simulink model "Controller_HIL"  (R2024a)
settings: Solver=FixedStepDiscrete  StartTime=0.0  StopTime=inf  FixedStep=ts_controller  RelTol=1e-3
InitFcn:
  | mbd_s32k_consistency_checks(bdroot(gcs));
undefined symbols (not defined in the file): Battery, BMS_Controller_State, Charging_State, currentFactor, CV_Gain, DiscIntNeverNeededParam, I_cc, LQFP, MaxCellVoltThrsld, noCurrent, Ns_Module, NumModules, OverCellVoltageLimit, SOCInit, SRE, ts_controller, ts_system, UnderCellVoltageLimit, voltThreshold
libraries: mbd_s32k1xx_ec_toolbox x104, etargetslib x95, mbd_bcc_ec_toolbox x30, hdlsllib x11, simulink x6, sharedTrackingLibrary x2
(part 1 of 4)
settings Model: DataDictionary=VTOLDynamicsData.sldd  EnableAccessToBaseWorkspace=off  Creator=vasileios.amoiridis  LastModifiedBy=jatin.anand
settings DataIOCC: ExternalInput=off  InitialState=off  SaveOutput=off  SignalLogging=off  SaveTime=off
settings OptimizationCC: DefaultParameterBehavior=Inlined  DefaultUnderspecifiedDataType=single  EnhancedBackFolding=on  PassReuseOutputArgsAs=Individual arguments  ZeroExternalMemoryAtStartup=off  ZeroInternalMemoryAtStartup=off  OptimizeBlockOrder=speed  DifferentSizesBufferReuse=on  OptimizationCustomize=off  EfficientTunableParamExpr=on
settings DebuggingCC: InheritedTsInSrcMsg=none  SingleTaskRateTransMsg=error  ParameterTunabilityLossMsg=error  UnconnectedInputMsg=error  UnconnectedOutputMsg=error  UnconnectedLineMsg=error  UnknownTsInhSupMsg=error
settings HardwareCC: ProdBitPerPointer=32  ProdBitPerSizeT=32  ProdBitPerPtrDiffT=32  ProdLargestAtomicInteger=Long  ProdLargestAtomicFloat=Double  ProdWordSize=32  ProdHWDeviceType=ARM Compatible->ARM Cortex
settings SFSimCC: MATLABDynamicMemAlloc=off
settings RTWCC: Description=Model Based Design Toolbox S32K1xx Code Generation Target  SystemTargetFile=mbd_s32k.tlc  MakeCommand=mbd_s32k_make_rtw COPY_MDLREF_INCLUDES=0  TemplateMakefile=mbd_s32k.tmf  GPUComputeCapability=3.5
settings CodeAppCC: ForceParamTrailComments=on  IgnoreCustomStorageClasses=off  OperatorAnnotations=on  SimulinkDataObjDesc=on  SFDataObjDesc=on  InsertBlockDesc=on
settings STFCustomTargetCC: MultiwordLength=256  CombineOutputUpdateFcns=on  ERTCustomFileBanners=on  SupportContinuousTime=off  SupportNonInlinedSFcns=off  RemoveResetFunc=on  MATLABClassNameForMDSCustomization=Simulink.SoftwareTarget.ERTCustomization  GRTInterface=off  UseToolchainInfoCompliant=off  SystemTargetFile=mbd_s32k.tlc
settings ERTTargetCC: TargetLangStandard=C99 (ISO)  ParMdlRefBuildCompliant=off  CompOptLevelCompliant=off  ConcurrentExecutionCompliant=off  ModelStepFunctionPrototypeControlCompliant=off  CPPClassGenCompliant=off  UseToolchainInfoCompliant=off  InlinedParameterPlacement=NonHierarchical  ERTSrcFileBannerTemplate=mbd_ert_code_template.cgt  ERTHdrFileBannerTemplate=mbd_ert_code_template.cgt  ERTDataSrcFileTemplate=mbd_ert_code_template.cgt  ERTDataHdrFileTemplate=mbd_ert_code_template.cgt  ERTCustomFileTemplate=example_file_process.tlc

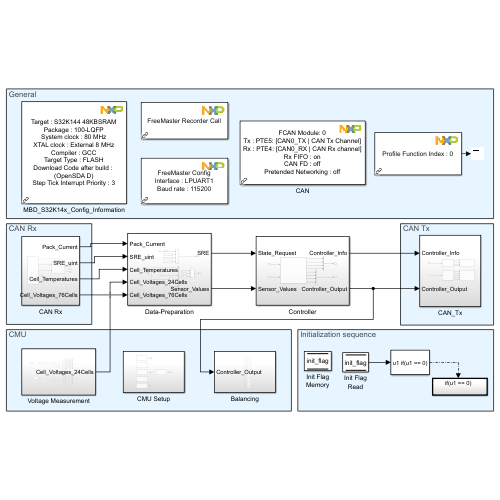
[thumbnail: Simulink's stored preview of the top-level diagram]
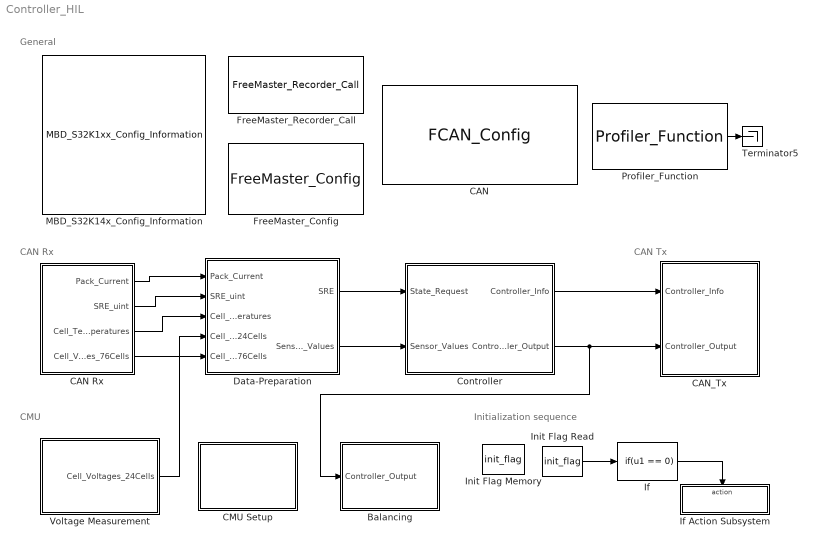
== system Controller_HIL ==
  note: CAN Tx
  note: CAN Rx
  note: CMU
  note: General
  note: Initialization sequence
  Balancing : Subsystem
  CAN : mbd_s32k1xx_ec_toolbox/Communication Blocks/CAN Blocks/FCAN_Config  Priority=1  can_instance=0  can_mode=Normal mode  can_max_num_mb=32  can_rx=PTE4: [CAN0_RX | CAN Rx channel]  can_tx=PTE5: [CAN0_TX | CAN Tx Channel]  show_adv_opts=on  can_clk_src=Peripheral clock  can_clk_freq=80 MHz  bitrate_to_time_seg=on  bitrate=1000  sample_point=80  real_bitrate=1000  real_sample_point=80  prop_delay=250  bus_length=1  tq=100.0  time_quanta=10  can_presdiv=8  can_propseg=6  can_pseg1=1  can_pseg2=2  can_rjw=1  cbt_bitrate=2000  cbt_sample_point=87.5  cbt_real_bitrate=2000  cbt_real_sample_point=80  cbt_tq=12.5  cbt_time_quanta=40  can_cbt_presdiv=1  can_cbt_propseg=29  can_cbt_pseg1=5  can_cbt_pseg2=5  can_cbt_rjw=5  can_fd_enable=off  can_payload=8  tdc_enable=off  tdc_offset=20  can_rxfifo_enable=on  can_num_id_filters=16  can_fifo_id_format=A  can_fifo_id_filter={{false,false,'0x401'},{false,false,'0x402'},{false,false,'0x403'},{false,false,'0x404'},{false,false,'0x405'},{false,false,'0x406'},{false,false,'0x407'},{false,false,'0x408'},{false,false,'0x409'},{false,false,'0x0'},{false,false,'0x0'},{false,false,'0x0'},{false,false,'0x0'},{false,false,'0x0'},{false,false,'0x0'},{false,false,'0x0'}}  can_pn_enable=off  can_wakeup_match=off  can_wakeup_timeout=off  can_timeout_en=off  can_match_timeout=1  can_multiple_matches_en=off  can_num_matches=1  can_idfilter_extendedid=off  can_idfilter_remoteframe=off  can_idfilter_type=Match exact  can_idfilter_id1=0  can_idfilter_id2=0  can_payloadfilter_enable=off  can_payloadfilter_dlclow=0  can_payloadfilter_dlchigh=0  can_payloadfilter_type=Match exact  can_payloadfilter_payload1_b0=0  can_payloadfilter_payload1_b1=0  can_payloadfilter_payload1_b2=0  can_payloadfilter_payload1_b3=0  can_payloadfilter_payload1_b4=0  can_payloadfilter_payload1_b5=0  can_payloadfilter_payload1_b6=0  can_payloadfilter_payload1_b7=0  can_payloadfilter_payload2_b0=0  can_payloadfilter_payload2_b1=0  can_payloadfilter_payload2_b2=0  can_payloadfilter_payload2_b3=0  can_payloadfilter_payload2_b4=0  can_payloadfilter_payload2_b5=0  can_payloadfilter_payload2_b6=0  can_payloadfilter_payload2_b7=0
  CAN Rx : Subsystem
  CAN_Tx : Subsystem
  CMU Setup : Subsystem
  Controller : Subsystem
  Data-Preparation : Subsystem
  FreeMaster_Config : mbd_s32k1xx_ec_toolbox/Utility Blocks/FreeMaster_Config  interface=LPUART1  baudrate=115200  rxd=PTC6: [LPUART1_RX | Receive]  txd=PTC7: [LPUART1_TX | Transmit]  mode=Short Interrupt  isr_prio=1  show_adv_opts=on  use_scope=on  max_scope_vars=8  use_recorder=on  max_rec_vars=8  rec_buff_size=512  rec_timebase=100 milliseconds  comm_buffer_size_auto=on  comm_buffer_size=255  comm_rqueue_size_default=on  comm_rqueue_size=32
  FreeMaster_Recorder_Call : mbd_s32k1xx_ec_toolbox/Utility Blocks/FreeMaster_Recorder_Call
  If : If  IfExpression=u1 == 0  ShowElse=off
  If Action Subsystem : Subsystem  TreatAsAtomicUnit=on
  Init Flag Memory : DataStoreMemory  DataStoreName=init_flag  ReadBeforeWriteMsg=warning  WriteAfterWriteMsg=warning  WriteAfterReadMsg=warning  ShowAdditionalParam=off  OutDataTypeStr=uint32
  Init Flag Read : DataStoreRead  DataStoreName=init_flag  IndexOptions=Index vector (dialog)  Indices=1  OutputSizes=1
  MBD_S32K14x_Config_Information : mbd_s32k1xx_ec_toolbox/MBD_S32K1xx_Config_Information  Priority=0  mbdt_ver=0  disp_str=|  config_params=[]  mcu_target_name=S32K144  mcu_target_package=100-LQFP  mcu_target_sram_size=48KB  mcu_system_clock_freq=80  mcu_xtal_freq=External 8  mcu_steptick_timer=LPIT Channel 0  mcu_steptick_prio=3  ds_import_enable=on  target_compiler=GCC  target_memory=FLASH  gcc_target_compile_opts=-mthumb -mfloat-abi=hard -mfpu=fpv4-sp-d16 -O1 -g -gstrict-dwarf  gcc_target_assemble_opts=-mthumb -mfloat-abi=hard -mfpu=fpv4-sp-d16 -g  gcc_target_link_opts=-mthumb -mfloat-abi=hard -mfpu=fpv4-sp-d16  gcc_target_default_lcf=on  gcc_target_user_lcf=S32K144_48_flash.ld  ghs_target_compile_opts=-cpu=cortexm4f -thumb -DARM_MATH_CM4 -fpu=vfpv4_d16 -fsingle -Ogeneral -Wundef -Wimplicit-int -Wshadow -Wtrigraphs --no_commons --gnu_asm -gnu99 -gdwarf-2 -G  ghs_target_assemble_opts=-cpu=cortexm4f -fpu=vfpv4_d16  ghs_target_link_opts=-cpu=cortexm4f -thumb -fpu=vfpv4_d16  ghs_target_default_lcf=off  ghs_target_user_lcf=S32K144_48_flash.ld  iar_target_compile_opts=--cpu=Cortex-M4F --thumb --fpu=VFPv4_sp -Ol -e --debug --dlib_config normal  iar_target_assemble_opts=--cpu Cortex-M4F --thumb --fpu VFPv4_sp  iar_target_link_opts=--no_exceptions --vfe --inline  iar_target_default_lcf=off  iar_target_user_lcf=S32K144_48_flash.icf  pil_download_enable=off  rbl_download_enable=on  rbl_start_delay=5000000  rbl_download_interface=OpenSDA  rbl_restart_request=off  rbl_com_port=Custom  rbl_com_port_custom=COM1  pil_download_rate=57600  pil_download_rate_custom=115200  pil_opensda_drive=Custom  pil_opensda_drive_custom=D  jtag_interface=OpenSDA Embedded Debug  jlink_default_path=on  jlink_user_path=C:\Program Files\SEGGER\JLink\  pil_uart_instance=1  pil_uart_rx=PTC6: [LPUART1_RX | Receive]  pil_uart_tx=PTC7: [LPUART1_TX | Transmit]  FTM_PWM_PcrCheckEnDis=on  FTM_Input_Edge_Inputs_PcrCheckEnDis=on  FTM_Dual_Edge_Inputs_PcrCheckEnDis=on  FTM_Quadrature_Inputs_PcrCheckEnDis=on  FTM_Hall_Sensor_Inputs_PcrCheckEnDis=on  LPTMR_PcrCheckEnDis=on  PIT_PcrCheckEnDis=on  RTC_PcrCheckEnDis=on  FlexCAN_PcrCheckEnDis=on  LIN_PcrCheckEnDis=on  FlexIO_PcrCheckEnDis=on  LPI2C_PcrCheckEnDis=on  LPSPI_PcrCheckEnDis=on  LPUART_PcrCheckEnDis=on  CMP_PcrCheckEnDis=on  GPIO_OutputPcrCheckEnDis=on  GPIO_InputPcrCheckEnDis=on  SBC_PcrCheckEnDis=on  BMS_PcrCheckEnDis=on  AMMCLIB_PcrCheckEnDis=on  FM_PcrCheckEnDis=on  Profile_PcrCheckEnDis=on  ConfigParams_PcrCheckEnDis=on  ModelRef_PcrCheckEnDis=on  PDB0_PcrCheckEnDis=on  CSEc_PcrCheckEnDis=on  eDMA_PcrCheckEnDis=on  FLASH_PcrCheckEnDis=on  ADC_PcrCheckEnDis=on  WDOG_PcrCheckEnDis=on
      | Target : S32K144-64KB_SRAM
      | Package : 100-pin
      | System clock : 80 MHz
      | XTAL clock : External 8 MHz
      | Compiler : GCC
      | Target Type : FLASH
      | Download Code after build : (OpenSDA: E)
      | Step Tick Interrupt Priority : 15
  Profiler_Function : mbd_s32k1xx_ec_toolbox/Utility Blocks/Profiler_Function  profile_indx=0
      settings: showOut=on
  Terminator5 : Terminator
  Voltage Measurement : Subsystem
  wires:
  Controller/2(Controller_Output) -> Balancing/1(Controller_Output), CAN_Tx/2(Controller_Output)
  Profiler_Function/1 -> Terminator5/1
  Data-Preparation/2(Sensor_Values) -> Controller/2(Sensor_Values)
  Controller/1(Controller_Info) -> CAN_Tx/1(Controller_Info)
  If/1 -> If Action Subsystem/Action
  Data-Preparation/1(SRE) -> Controller/1(State_Request)
  Init Flag Read/1 -> If/1
  CAN Rx/1(Pack_Current) -> Data-Preparation/1(Pack_Current)
  CAN Rx/2(SRE_uint) -> Data-Preparation/2(SRE_uint)
  CAN Rx/3(Cell_Temperatures) -> Data-Preparation/3(Cell_Temperatures)
  Voltage Measurement/1(Cell_Voltages_24Cells) -> Data-Preparation/4(Cell_Voltages_24Cells)
  CAN Rx/4(Cell_Voltages_76Cells) -> Data-Preparation/5(Cell_Voltages_76Cells)

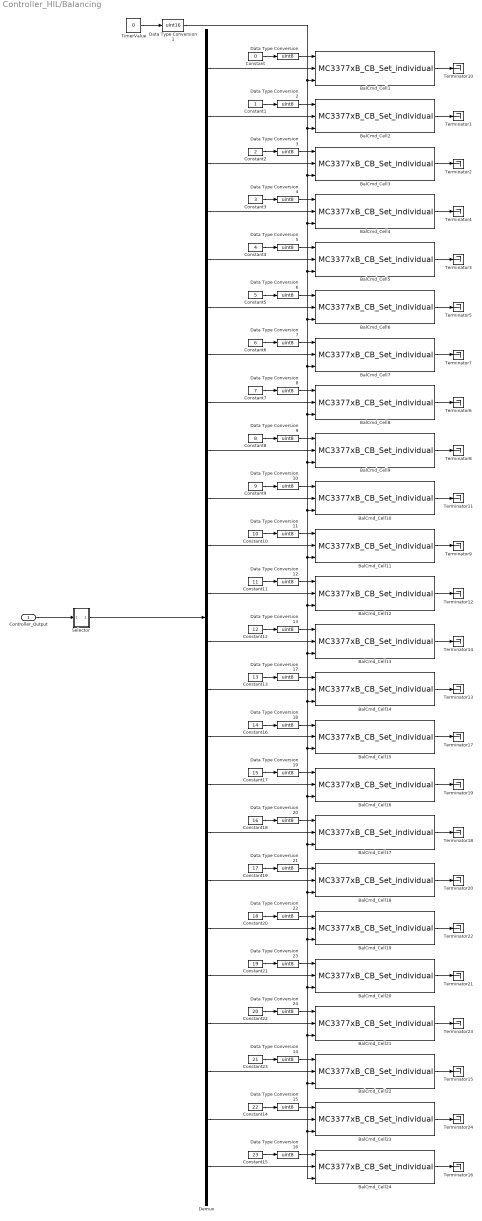
== system Controller_HIL/Balancing ==
  Controller_Output : Inport
  BalCmd_Cell{1..12} (12 alike) : mbd_bcc_ec_toolbox/BMS/MC3377xB_CB_Set_individual  bccInstance=0  bccCID=1
  BalCmd_Cell{13..24} (12 alike) : mbd_bcc_ec_toolbox/BMS/MC3377xB_CB_Set_individual  bccInstance=0  bccCID=2
  Constant : Constant  Value=0  SampleTime=-1
  Constant1 : Constant  SampleTime=-1
  Constant10 : Constant  Value=10  SampleTime=-1
  Constant11 : Constant  Value=11  SampleTime=-1
  Constant12 : Constant  Value=12  SampleTime=-1
  Constant13 : Constant  Value=13  SampleTime=-1
  Constant14 : Constant  Value=22  SampleTime=-1
  Constant15 : Constant  Value=23  SampleTime=-1
  Constant16 : Constant  Value=14  SampleTime=-1
  Constant17 : Constant  Value=15  SampleTime=-1
  Constant18 : Constant  Value=16  SampleTime=-1
  Constant19 : Constant  Value=17  SampleTime=-1
  Constant2 : Constant  Value=2  SampleTime=-1
  Constant20 : Constant  Value=18  SampleTime=-1
  Constant21 : Constant  Value=19  SampleTime=-1
  Constant22 : Constant  Value=20  SampleTime=-1
  Constant23 : Constant  Value=21  SampleTime=-1
  Constant3 : Constant  Value=3  SampleTime=-1
  Constant4 : Constant  Value=4  SampleTime=-1
  Constant5 : Constant  Value=5  SampleTime=-1
  Constant6 : Constant  Value=6  SampleTime=-1
  Constant7 : Constant  Value=7  SampleTime=-1
  Constant8 : Constant  Value=8  SampleTime=-1
  Constant9 : Constant  Value=9  SampleTime=-1
  Data Type Conversion{,2..24} (24 alike) : DataTypeConversion  OutDataTypeStr=uint8  SaturateOnIntegerOverflow=off  RndMeth=Floor
  Data Type Conversion1 : DataTypeConversion  OutDataTypeStr=uint16  SaturateOnIntegerOverflow=off  RndMeth=Floor
  Demux : Demux  Outputs=24
  Selector : Subsystem
  Terminator{1..24} (24 alike) : Terminator
  TimerValue : Constant  Value=0  SampleTime=-1
  wires:
  Demux/12 -> BalCmd_Cell12/2
  Demux/3 -> BalCmd_Cell3/2
  BalCmd_Cell6/1 -> Terminator5/1
  Constant10/1 -> Data Type Conversion11/1
  Demux/10 -> BalCmd_Cell10/2
  BalCmd_Cell10/1 -> Terminator11/1
  Data Type Conversion6/1 -> BalCmd_Cell6/1
  Demux/1 -> BalCmd_Cell1/2
  Demux/5 -> BalCmd_Cell5/2
  Constant8/1 -> Data Type Conversion9/1
  Constant11/1 -> Data Type Conversion12/1
  TimerValue/1 -> Data Type Conversion1/1
  Constant6/1 -> Data Type Conversion7/1
  Data Type Conversion8/1 -> BalCmd_Cell8/1
  Data Type Conversion9/1 -> BalCmd_Cell9/1
  Data Type Conversion5/1 -> BalCmd_Cell5/1
  Constant9/1 -> Data Type Conversion10/1
  Selector/1(Out1) -> Demux/1
  Demux/11 -> BalCmd_Cell11/2
  Demux/9 -> BalCmd_Cell9/2
  BalCmd_Cell7/1 -> Terminator7/1
  Demux/8 -> BalCmd_Cell8/2
  Demux/2 -> BalCmd_Cell2/2
  Demux/7 -> BalCmd_Cell7/2
  Data Type Conversion11/1 -> BalCmd_Cell11/1
  Constant7/1 -> Data Type Conversion8/1
  Constant/1 -> Data Type Conversion/1
  BalCmd_Cell12/1 -> Terminator12/1
  Data Type Conversion7/1 -> BalCmd_Cell7/1
  Data Type Conversion10/1 -> BalCmd_Cell10/1
  BalCmd_Cell5/1 -> Terminator3/1
  BalCmd_Cell8/1 -> Terminator6/1
  Demux/4 -> BalCmd_Cell4/2
  Demux/6 -> BalCmd_Cell6/2
  BalCmd_Cell3/1 -> Terminator2/1
  Controller_Output/1 -> Selector/1(In1)
  Data Type Conversion12/1 -> BalCmd_Cell12/1
  Constant3/1 -> Data Type Conversion4/1
  Constant1/1 -> Data Type Conversion2/1
  BalCmd_Cell1/1 -> Terminator10/1
  BalCmd_Cell2/1 -> Terminator1/1
  Constant2/1 -> Data Type Conversion3/1
  Data Type Conversion/1 -> BalCmd_Cell1/1
  BalCmd_Cell4/1 -> Terminator4/1
  BalCmd_Cell9/1 -> Terminator8/1
  Constant5/1 -> Data Type Conversion6/1
  Data Type Conversion3/1 -> BalCmd_Cell3/1
  Data Type Conversion2/1 -> BalCmd_Cell2/1
  Data Type Conversion4/1 -> BalCmd_Cell4/1
  BalCmd_Cell11/1 -> Terminator9/1
  Constant4/1 -> Data Type Conversion5/1
  Constant17/1 -> Data Type Conversion19/1
  Constant18/1 -> Data Type Conversion20/1
  Data Type Conversion14/1 -> BalCmd_Cell22/1
  BalCmd_Cell23/1 -> Terminator24/1
  Data Type Conversion19/1 -> BalCmd_Cell16/1
  BalCmd_Cell21/1 -> Terminator23/1
  BalCmd_Cell13/1 -> Terminator14/1
  Constant14/1 -> Data Type Conversion15/1
  Constant16/1 -> Data Type Conversion18/1
  Data Type Conversion13/1 -> BalCmd_Cell13/1
  BalCmd_Cell19/1 -> Terminator22/1
  BalCmd_Cell14/1 -> Terminator13/1
  Data Type Conversion16/1 -> BalCmd_Cell24/1
  BalCmd_Cell15/1 -> Terminator17/1
  Constant19/1 -> Data Type Conversion21/1
  BalCmd_Cell16/1 -> Terminator19/1
  Data Type Conversion17/1 -> BalCmd_Cell14/1
  Data Type Conversion1/1 -> BalCmd_Cell5/3, BalCmd_Cell11/3, BalCmd_Cell17/3, BalCmd_Cell23/3, BalCmd_Cell24/3, BalCmd_Cell22/3, BalCmd_Cell21/3, BalCmd_Cell20/3, BalCmd_Cell19/3, BalCmd_Cell18/3, BalCmd_Cell16/3, BalCmd_Cell15/3, BalCmd_Cell14/3, BalCmd_Cell13/3, BalCmd_Cell12/3, BalCmd_Cell10/3, BalCmd_Cell9/3, BalCmd_Cell8/3, BalCmd_Cell7/3, BalCmd_Cell6/3, BalCmd_Cell4/3, BalCmd_Cell3/3, BalCmd_Cell2/3, BalCmd_Cell1/3
  Data Type Conversion24/1 -> BalCmd_Cell21/1
  Constant12/1 -> Data Type Conversion13/1
  BalCmd_Cell18/1 -> Terminator20/1
  Constant13/1 -> Data Type Conversion17/1
  BalCmd_Cell20/1 -> Terminator21/1
  BalCmd_Cell24/1 -> Terminator16/1
  BalCmd_Cell17/1 -> Terminator18/1
  Data Type Conversion22/1 -> BalCmd_Cell19/1
  BalCmd_Cell22/1 -> Terminator15/1
  Constant20/1 -> Data Type Conversion22/1
  Constant21/1 -> Data Type Conversion23/1
  Data Type Conversion15/1 -> BalCmd_Cell23/1
  Constant23/1 -> Data Type Conversion14/1
  Data Type Conversion20/1 -> BalCmd_Cell17/1
  Data Type Conversion23/1 -> BalCmd_Cell20/1
  Constant15/1 -> Data Type Conversion16/1
  Data Type Conversion21/1 -> BalCmd_Cell18/1
  Constant22/1 -> Data Type Conversion24/1
  Data Type Conversion18/1 -> BalCmd_Cell15/1
  Demux/13 -> BalCmd_Cell13/2
  Demux/14 -> BalCmd_Cell14/2
  Demux/15 -> BalCmd_Cell15/2
  Demux/16 -> BalCmd_Cell16/2
  Demux/17 -> BalCmd_Cell17/2
  Demux/18 -> BalCmd_Cell18/2
  Demux/19 -> BalCmd_Cell19/2
  Demux/20 -> BalCmd_Cell20/2
  Demux/21 -> BalCmd_Cell21/2
  Demux/22 -> BalCmd_Cell22/2
  Demux/23 -> BalCmd_Cell23/2
  Demux/24 -> BalCmd_Cell24/2

== system Controller_HIL/CAN Rx ==
  FCAN_Rx_FIFO_Complete_Isr : mbd_s32k1xx_ec_toolbox/Communication Blocks/CAN Blocks/FCAN_Isr  can_instance=0  can_event=Rx FIFO Complete
  RX_FIFO_Complete_Event : Subsystem
  Terminator : Terminator
  Terminator1 : Terminator
  Pack_Current : Outport
  SRE_uint : Outport  Port=2
  Cell_Temperatures : Outport  Port=3
  Cell_Voltages_76Cells : Outport  Port=4
  wires:
  FCAN_Rx_FIFO_Complete_Isr/4 -> Terminator/1
  FCAN_Rx_FIFO_Complete_Isr/5 -> Terminator1/1
  FCAN_Rx_FIFO_Complete_Isr/2 -> RX_FIFO_Complete_Event/1(ID)
  FCAN_Rx_FIFO_Complete_Isr/3 -> RX_FIFO_Complete_Event/2(Data)
  FCAN_Rx_FIFO_Complete_Isr/1 -> RX_FIFO_Complete_Event/Trigger
  RX_FIFO_Complete_Event/1(Pack_Current) -> Pack_Current/1
  RX_FIFO_Complete_Event/2(SRE_uint) -> SRE_uint/1
  RX_FIFO_Complete_Event/3(Cell_Temperatures) -> Cell_Temperatures/1
  RX_FIFO_Complete_Event/4(Cell_Voltages_76Cells) -> Cell_Voltages_76Cells/1

== system Controller_HIL/CAN_Tx ==
  Controller_Info : Inport
  Controller_Output : Inport  Port=2
  CAN_Data : Subsystem
  CAN_Data_HIL : Subsystem
  TX_Complete_HIL : Subsystem  TreatAsAtomicUnit=on
  Tx_Complete : Subsystem  TreatAsAtomicUnit=on
  wires:
  CAN_Data/4(Length_0x202) -> Tx_Complete/4(Length_0x202)
  CAN_Data/3(Data_0x202) -> Tx_Complete/3(Data_0x202)
  CAN_Data/1(Data_0x201) -> Tx_Complete/1(Data_0x201)
  CAN_Data/2(Length_0x201) -> Tx_Complete/2(Length_0x201)
  CAN_Data_HIL/1(Data_0x501) -> TX_Complete_HIL/1(Data_0x501)
  CAN_Data_HIL/2(Length_0x501) -> TX_Complete_HIL/2(Length_0x501)
  CAN_Data_HIL/4(Length_0x502) -> TX_Complete_HIL/4(Length_0x502)
  CAN_Data_HIL/3(Data_0x502) -> TX_Complete_HIL/3(Data_0x502)
  Controller_Info/1 -> CAN_Data_HIL/1(Controller_Info)
  Controller_Output/1 -> CAN_Data/1(Controller_Output)
  CAN_Data/5(Bal_Cmd_CAN) -> Tx_Complete/5(Bal_Cmd_CAN)

== system Controller_HIL/CMU Setup ==
  "LPSPI_RX " : mbd_s32k1xx_ec_toolbox/Communication Blocks/SPI Blocks/LPSPI_Config   InstanceNumber=0  Role=Slave  BaudRate=1000000  ShowAdvanced=on  sin=PTB3: [LPSPI0_SIN | LPSPI Serial Data Input]  sout=None  sck=PTB2: [LPSPI0_SCK | LPSPI Serial Clock I/O]  pcs0=None  pcs1=PTB5: [LPSPI0_PCS1 | Peripheral Chip Select 1]  pcs2=None  pcs3=None  CPHA=1  CPOL=0  BitOrder=MSB first  TransferSize=40  WhichPCS=1  PCSPol=ActiveLow  ContinuousTransfer=off
  LPSPI_TX : mbd_s32k1xx_ec_toolbox/Communication Blocks/SPI Blocks/LPSPI_Config   InstanceNumber=1  Role=Master  BaudRate=2000000  ShowAdvanced=on  sin=None  sout=PTB16: [LPSPI1_SOUT | LPSPI Serial Data Output]  sck=PTB14: [LPSPI1_SCK | LPSPI Serial Clock I/O]  pcs0=PTD3: [LPSPI1_PCS0 | Peripheral Chip Select 0]  pcs1=PTA6: [LPSPI1_PCS1 | Peripheral Chip Select 1]  pcs2=None  pcs3=None  CPHA=1  CPOL=0  BitOrder=MSB first  TransferSize=40  WhichPCS=1  PCSPol=ActiveLow  ContinuousTransfer=off
  MC3377xB_CB_Disable_Enable : mbd_bcc_ec_toolbox/BMS/MC3377xB_CB_Disable_Enable  bccInstance=0  bccCID=1  bccAction=Enable
  MC3377xB_CB_Disable_Enable1 : mbd_bcc_ec_toolbox/BMS/MC3377xB_CB_Disable_Enable  bccInstance=0  bccCID=2  bccAction=Enable
  MC3377xB_Config : mbd_bcc_ec_toolbox/BMS/MC3377xB_Config  Priority=1  bccInstance=0  bccMode=TPL  bccTPLDevNr=2  bccSpiDev=MC33771B  bccSpiCell=3  bccTPLDev1=MC33771B  bccTPLCell1=14  bccTPLDev2=MC33771B  bccTPLCell2=14  bccTPLDev3=MC33771B  bccTPLCell3=3  bccTPLDev4=MC33771B  bccTPLCell4=3  bccTPLDev5=MC33771B  bccTPLCell5=3  bccTPLDev6=MC33771B  bccTPLCell6=3  bccTPLDev7=MC33771B  bccTPLCell7=3  bccTPLDev8=MC33771B  bccTPLCell8=3  bccTPLDev9=MC33771B  bccTPLCell9=3  bccTPLDev10=MC33771B  bccTPLCell10=3  bccTPLDev11=MC33771B  bccTPLCell11=3  bccTPLDev12=MC33771B  bccTPLCell12=3  bccTPLDev13=MC33771B  bccTPLCell13=3  bccTPLDev14=MC33771B  bccTPLCell14=3  bccTPLDev15=MC33771B  bccTPLCell15=3  bccSpiMaster=1  bccSPIMasterCSCustom=off  bccSPIMasterPCS=LPSPI_PCS1  bccSPIMasterPCSGPIO=PTA0: [PTA0 | Port A I/O]  bccSpiSlave=0  bccSPISlavePCS=LPSPI_PCS1  bccSPI_RESET_ALT0=PTA0: [PTA0 | Port A I/O]  bccTPL_ENABLE=PTB0: [PTB0 | Port B I/O]  bccTPL_INTB=PTB1: [PTB1 | Port B I/O]  bccNTCBeta=3900  bccNTCRes=6800  bccNTCRefR=10000  bccNTCRefT=25  bccShunt=10000
  MC3377xB_Start_Conversion : mbd_bcc_ec_toolbox/BMS/MC3377xB_Start_Conversion  Priority=100  bccInstance=0  bccCID=1  bccCIDGlobal=on  bccADCCFG=0
  Terminator{,1..3} (4 alike) : Terminator
  wires:
  MC3377xB_CB_Disable_Enable/1 -> Terminator/1
  MC3377xB_Config/1 -> Terminator2/1
  MC3377xB_Start_Conversion/1 -> Terminator1/1
  MC3377xB_CB_Disable_Enable1/1 -> Terminator3/1

== system Controller_HIL/Controller ==
  State_Request : Inport  OutDataTypeStr=Enum: SRE  PortDimensions=1
  Sensor_Values : Inport  Port=2  OutDataTypeStr=Bus: Sensor_Values  BusOutputAsStruct=on
  Bus Creator : BusCreator  Inputs=4  OutDataTypeStr=Bus: Controller_Info
  Bus Creator1 : BusCreator  Inputs=4  OutDataTypeStr=Bus: Controller_Output  NonVirtualBus=on
      settings: InheritFromInputs=off
  Controller : Subsystem
  Controller_Info : Outport
  Controller_Output : Outport  Port=2  OutDataTypeStr=Bus: Controller_Output  VectorParamsAs1DForOutWhenUnconnected=off  BusOutputAsStruct=on
  wires:
  Sensor_Values/1 -> Controller/1(Sensor_Values)
  Controller/8(Bal_Cmd) -> Bus Creator1/4
  Controller/5(Discharge_Current_Limit) -> Bus Creator1/1
  Controller/6(Charge_Current_Limit) -> Bus Creator1/2
  Bus Creator1/1 -> Controller_Output/1  "Controller_Output"
  Bus Creator/1 -> Controller_Info/1  "Controller_Info"
  State_Request/1 -> Controller/2(State_Request)
  Controller/4(SOC) -> Bus Creator/4
  Controller/3(BMS_Controller_State) -> Bus Creator/3
  Controller/2(Charging_State) -> Bus Creator/2
  Controller/7(Charge_Current_Req) -> Bus Creator1/3
  Controller/1(Faults) -> Bus Creator/1

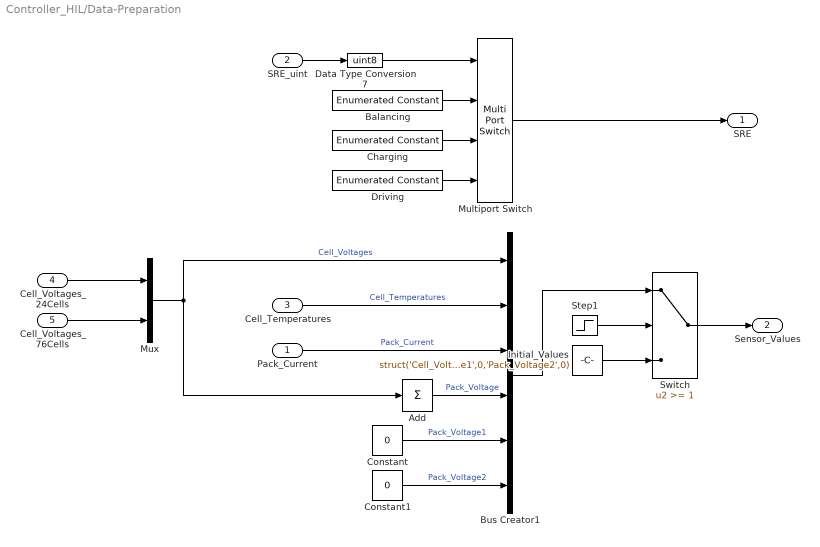
== system Controller_HIL/Data-Preparation ==
  Pack_Current : Inport
  SRE_uint : Inport  Port=2
  Cell_Temperatures : Inport  Port=3
  Cell_Voltages_24Cells : Inport  Port=4
  Cell_Voltages_76Cells : Inport  Port=5
  Add : Sum  Inputs=+
  Balancing : simulink/Sources/Enumerated Constant  OutDataTypeStr=Enum: SRE  Value=SRE.Standby  SampleTime=-1
  Bus Creator1 : BusCreator  Inputs=6  OutDataTypeStr=Bus: Sensor_Values  NonVirtualBus=on
  Charging : simulink/Sources/Enumerated Constant  OutDataTypeStr=Enum: SRE  Value=SRE.Flying  SampleTime=-1
  Constant : Constant  Value=0  OutDataTypeStr=single
  Constant1 : Constant  Value=0  OutDataTypeStr=single
  Data Type Conversion7 : DataTypeConversion  OutDataTypeStr=uint8  SaturateOnIntegerOverflow=off  RndMeth=Floor
  Driving : simulink/Sources/Enumerated Constant  OutDataTypeStr=Enum: SRE  Value=SRE.Charging  SampleTime=-1
  Initial_Values : Constant  Value=struct('Cell_Voltages',3.6*ones(1, Ns_Module*NumModules),'Cell_Temperatures',293.15*ones(1,Ns_Module*NumModules),'Pack_Current',0,'Pack_Voltage',3.6*Ns_Module*NumModules,'Pack_Voltage1',0,'Pack_Voltage2',0)  OutDataTypeStr=Bus: Sensor_Values  SampleTime=-1
  Multiport Switch : MultiPortSwitch  DataPortOrder=Zero-based contiguous  zeroidx=on  SaturateOnIntegerOverflow=off  InputSameDT=off
  Mux : Mux  Inputs=2
  Step1 : Step
  Switch : Switch  Threshold=1  SaturateOnIntegerOverflow=off  InputSameDT=off
  SRE : Outport
  Sensor_Values : Outport  Port=2
  wires:
  Bus Creator1/1 -> Switch/1
  Step1/1 -> Switch/2
  Pack_Current/1 -> Bus Creator1/3  "Pack_Current"
  Cell_Temperatures/1 -> Bus Creator1/2  "Cell_Temperatures"
  Multiport Switch/1 -> SRE/1
  Switch/1 -> Sensor_Values/1
  Driving/1 -> Multiport Switch/4
  Charging/1 -> Multiport Switch/3
  Balancing/1 -> Multiport Switch/2
  Data Type Conversion7/1 -> Multiport Switch/1
  Initial_Values/1 -> Switch/3
  Add/1 -> Bus Creator1/4  "Pack_Voltage"
  SRE_uint/1 -> Data Type Conversion7/1
  Cell_Voltages_24Cells/1 -> Mux/1
  Cell_Voltages_76Cells/1 -> Mux/2
  Mux/1 -> Bus Creator1/1, Add/1  "Cell_Voltages"
  Constant/1 -> Bus Creator1/5  "Pack_Voltage1"
  Constant1/1 -> Bus Creator1/6  "Pack_Voltage2"

== system Controller_HIL/If Action Subsystem ==
  Action Port : ActionPort  ActionPortLabel=if(u1 == 0)
  Constant : Constant  OutDataTypeStr=uint32  SampleTime=-1
  FCAN_Receive_FIFO : mbd_s32k1xx_ec_toolbox/Communication Blocks/CAN Blocks/FCAN_Receive  can_instance=0  can_mode=Non-blocking  can_timeout_ms=0  can_mb_idx=0  can_mb_init=Once  show_id_input=off  can_extended_id=off  can_is_remote=off  can_id=0x7FF  can_msg_mask=0  show_adv_opts=on  can_use_rxfifo=on  can_fd_enable=off
  Init Flag Write : DataStoreWrite  DataStoreName=init_flag  IndexOptions=Index vector (dialog)  Indices=1  OutputSizes=1
  wires:
  Constant/1 -> Init Flag Write/1

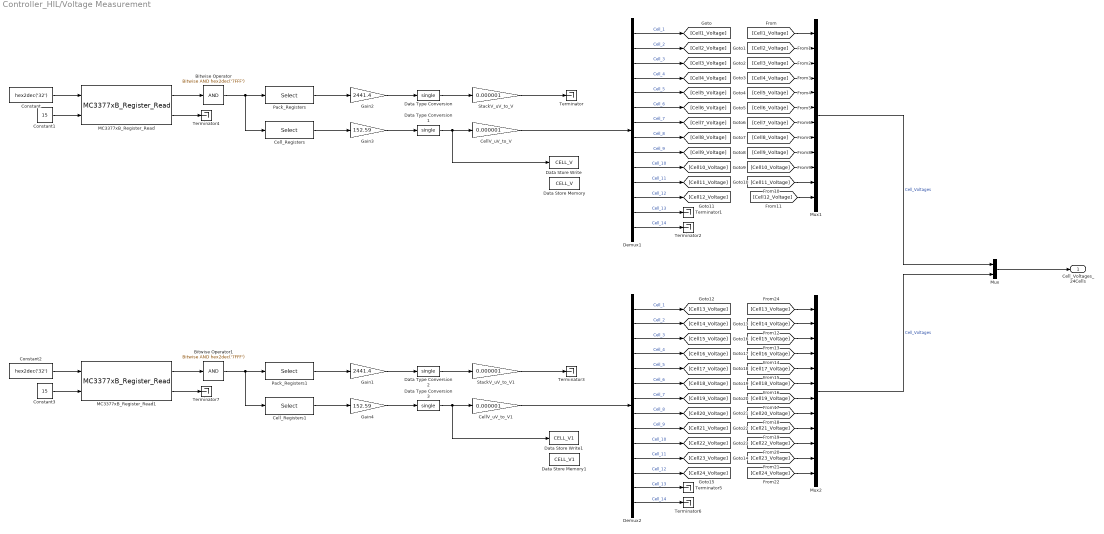
== system Controller_HIL/Voltage Measurement ==
  Bitwise Operator : simulink/Logic and Bit Operations/Bitwise Operator  logicop=AND  UseBitMask=on  BitMask=hex2dec('7FFF')  BitMaskRealWorld=Stored Integer
  Bitwise Operator1 : simulink/Logic and Bit Operations/Bitwise Operator  logicop=AND  UseBitMask=on  BitMask=hex2dec('7FFF')  BitMaskRealWorld=Stored Integer
  CellV_uV_to_V : Gain  Gain=0.000001
  CellV_uV_to_V1 : Gain  Gain=0.000001
  Cell_Registers : Selector  InputPortWidth=15  IndexOptions=Index vector (dialog)  Indices=[15 14 13 12 11 10 9 8 7 6 5 4 3 2]  OutputSizes=1
  Cell_Registers1 : Selector  InputPortWidth=15  IndexOptions=Index vector (dialog)  Indices=[15 14 13 12 11 10 9 8 7 6 5 4 3 2]  OutputSizes=1
  Constant : Constant  Value=hex2dec('32')  OutDataTypeStr=Inherit: Inherit via back propagation  SampleTime=-1
  Constant1 : Constant  Value=15  OutDataTypeStr=Inherit: Inherit via back propagation  SampleTime=-1
  Constant2 : Constant  Value=hex2dec('32')  OutDataTypeStr=Inherit: Inherit via back propagation  SampleTime=-1
  Constant3 : Constant  Value=15  OutDataTypeStr=Inherit: Inherit via back propagation  SampleTime=-1
  Data Store Memory : DataStoreMemory  DataStoreName=CELL_V  WriteAfterWriteMsg=warning  InitialValue=zeros(14,1)  ShowAdditionalParam=off
  Data Store Memory1 : DataStoreMemory  DataStoreName=CELL_V1  WriteAfterWriteMsg=warning  InitialValue=zeros(14,1)  ShowAdditionalParam=off
  Data Store Write : DataStoreWrite  DataStoreName=CELL_V  IndexOptions=Index vector (dialog)  Indices=1  OutputSizes=1
  Data Store Write1 : DataStoreWrite  DataStoreName=CELL_V1  IndexOptions=Index vector (dialog)  Indices=1  OutputSizes=1
  Data Type Conversion{,1..3} (4 alike) : DataTypeConversion  OutDataTypeStr=single  SaturateOnIntegerOverflow=off  RndMeth=Floor
  Demux1 : Demux  Outputs=14
  Demux2 : Demux  Outputs=14
  Gain1 : Gain  Gain=2441.4
  Gain2 : Gain  Gain=2441.4
  Gain3 : Gain  Gain=152.59
  Gain4 : Gain  Gain=152.59
  MC3377xB_Register_Read : mbd_bcc_ec_toolbox/BMS/MC3377xB_Register_Read  bccInstance=0  bccCID=1
  MC3377xB_Register_Read1 : mbd_bcc_ec_toolbox/BMS/MC3377xB_Register_Read  bccInstance=0  bccCID=2
  Mux : Mux  Inputs=2
  Mux1 : Mux  Inputs=12
  Mux2 : Mux  Inputs=12
  Pack_Registers : Selector  InputPortWidth=15  IndexOptions=Index vector (dialog)  Indices=[1]  OutputSizes=1
  Pack_Registers1 : Selector  InputPortWidth=15  IndexOptions=Index vector (dialog)  Indices=[1]  OutputSizes=1
  StackV_uV_to_V : Gain  Gain=0.000001
  StackV_uV_to_V1 : Gain  Gain=0.000001
  Terminator{,1..7} (8 alike) : Terminator
  Cell_Voltages_24Cells : Outport
  wires:
  Pack_Registers/1 -> Gain2/1
  Demux1/12 -> [Cell12_Voltage]  "Cell_12"
  CellV_uV_to_V/1 -> Demux1/1
  Demux1/13 -> Terminator1/1  "Cell_13"
  Demux1/10 -> [Cell10_Voltage]  "Cell_10"
  Demux1/2 -> [Cell2_Voltage]  "Cell_2"
  Demux1/14 -> Terminator2/1  "Cell_14"
  Demux1/7 -> [Cell7_Voltage]  "Cell_7"
  Constant1/1 -> MC3377xB_Register_Read/2
  Demux1/3 -> [Cell3_Voltage]  "Cell_3"
  Data Type Conversion1/1 -> Data Store Write/1, CellV_uV_to_V/1
  Demux1/11 -> [Cell11_Voltage]  "Cell_11"
  Demux1/9 -> [Cell9_Voltage]  "Cell_9"
  Gain2/1 -> Data Type Conversion/1
  Demux1/1 -> [Cell1_Voltage]  "Cell_1"
  Data Type Conversion/1 -> StackV_uV_to_V/1
  Bitwise Operator/1 -> Cell_Registers/1, Pack_Registers/1
  Cell_Registers/1 -> Gain3/1
  Demux1/6 -> [Cell6_Voltage]  "Cell_6"
  Gain3/1 -> Data Type Conversion1/1
  Demux1/5 -> [Cell5_Voltage]  "Cell_5"
  MC3377xB_Register_Read/1 -> Bitwise Operator/1
  Demux1/8 -> [Cell8_Voltage]  "Cell_8"
  Demux1/4 -> [Cell4_Voltage]  "Cell_4"
  StackV_uV_to_V/1 -> Terminator/1
  MC3377xB_Register_Read/2 -> Terminator4/1
  Constant/1 -> MC3377xB_Register_Read/1
  [Cell1_Voltage] -> Mux1/1
  [Cell2_Voltage] -> Mux1/2
  [Cell3_Voltage] -> Mux1/3
  [Cell10_Voltage] -> Mux1/10
  [Cell12_Voltage] -> Mux1/12
  [Cell4_Voltage] -> Mux1/4
  [Cell5_Voltage] -> Mux1/5
  [Cell6_Voltage] -> Mux1/6
  [Cell7_Voltage] -> Mux1/7
  [Cell8_Voltage] -> Mux1/8
  [Cell9_Voltage] -> Mux1/9
  [Cell11_Voltage] -> Mux1/11
  [Cell14_Voltage] -> Mux2/2
  StackV_uV_to_V1/1 -> Terminator3/1
  Demux2/4 -> [Cell16_Voltage]  "Cell_4"
  [Cell15_Voltage] -> Mux2/3
  Demux2/6 -> [Cell18_Voltage]  "Cell_6"
  Bitwise Operator1/1 -> Cell_Registers1/1, Pack_Registers1/1
  Demux2/8 -> [Cell20_Voltage]  "Cell_8"
  Data Type Conversion3/1 -> Data Store Write1/1, CellV_uV_to_V1/1
  Gain1/1 -> Data Type Conversion2/1
  Demux2/9 -> [Cell21_Voltage]  "Cell_9"
  MC3377xB_Register_Read1/2 -> Terminator7/1
  Demux2/5 -> [Cell17_Voltage]  "Cell_5"
  [Cell13_Voltage] -> Mux2/1
  Gain4/1 -> Data Type Conversion3/1
  Cell_Registers1/1 -> Gain4/1
  Demux2/1 -> [Cell13_Voltage]  "Cell_1"
  MC3377xB_Register_Read1/1 -> Bitwise Operator1/1
  Demux2/7 -> [Cell19_Voltage]  "Cell_7"
  Demux2/12 -> [Cell24_Voltage]  "Cell_12"
  CellV_uV_to_V1/1 -> Demux2/1
  Demux2/10 -> [Cell22_Voltage]  "Cell_10"
  Demux2/13 -> Terminator5/1  "Cell_13"
  Demux2/14 -> Terminator6/1  "Cell_14"
  Demux2/2 -> [Cell14_Voltage]  "Cell_2"
  Demux2/3 -> [Cell15_Voltage]  "Cell_3"
  Data Type Conversion2/1 -> StackV_uV_to_V1/1
  Pack_Registers1/1 -> Gain1/1
  Mux2/1 -> Mux/2  "Cell_Voltages"
  [Cell22_Voltage] -> Mux2/10
  [Cell19_Voltage] -> Mux2/7
  [Cell18_Voltage] -> Mux2/6
  [Cell20_Voltage] -> Mux2/8
  [Cell21_Voltage] -> Mux2/9
  [Cell17_Voltage] -> Mux2/5
  [Cell24_Voltage] -> Mux2/12
  [Cell16_Voltage] -> Mux2/4
  [Cell23_Voltage] -> Mux2/11
  Demux2/11 -> [Cell23_Voltage]  "Cell_11"
  Mux1/1 -> Mux/1  "Cell_Voltages"
  Mux/1 -> Cell_Voltages_24Cells/1
  Constant2/1 -> MC3377xB_Register_Read1/1
  Constant3/1 -> MC3377xB_Register_Read1/2

== system Controller_HIL/Balancing/Selector ==
  In1 : Inport
  Bus Creator : BusCreator  Inputs=24
  Bus Selector : BusSelector  OutputSignals=Bal_Cmd
  Demux : Demux  Outputs=100
  Mux1 : Mux  Inputs=76
  Terminator : Terminator
  Out1 : Outport
  wires:
  Demux/1 -> Bus Creator/1
  Demux/2 -> Bus Creator/2
  Demux/3 -> Bus Creator/3
  Demux/4 -> Bus Creator/4
  Demux/5 -> Bus Creator/5
  Demux/6 -> Bus Creator/6
  Demux/7 -> Bus Creator/7
  Demux/8 -> Bus Creator/8
  Demux/9 -> Bus Creator/9
  Demux/10 -> Bus Creator/10
  Demux/11 -> Bus Creator/11
  Demux/12 -> Bus Creator/12
  Demux/13 -> Bus Creator/13
  Demux/14 -> Bus Creator/14
  Demux/15 -> Bus Creator/15
  Demux/16 -> Bus Creator/16
  Demux/17 -> Bus Creator/17
  Demux/18 -> Bus Creator/18
  Demux/19 -> Bus Creator/19
  Demux/20 -> Bus Creator/20
  Demux/21 -> Bus Creator/21
  Demux/22 -> Bus Creator/22
  Demux/23 -> Bus Creator/23
  Demux/24 -> Bus Creator/24
  Bus Creator/1 -> Out1/1
  Demux/25 -> Mux1/1
  Demux/26 -> Mux1/2
  Demux/27 -> Mux1/3
  Demux/28 -> Mux1/4
  Demux/29 -> Mux1/5
  Demux/30 -> Mux1/6
  Demux/31 -> Mux1/7
  Demux/32 -> Mux1/8
  Demux/33 -> Mux1/9
  Demux/34 -> Mux1/10
  Demux/35 -> Mux1/11
  Demux/36 -> Mux1/12
  Demux/37 -> Mux1/13
  Demux/38 -> Mux1/14
  Demux/39 -> Mux1/15
  Demux/40 -> Mux1/16
  Demux/41 -> Mux1/17
  Demux/42 -> Mux1/18
  Demux/43 -> Mux1/19
  Demux/44 -> Mux1/20
  Demux/45 -> Mux1/21
  Demux/46 -> Mux1/22
  Demux/47 -> Mux1/23
  Demux/48 -> Mux1/24
  Demux/49 -> Mux1/25
  Demux/50 -> Mux1/26
  Demux/51 -> Mux1/27
  Demux/52 -> Mux1/28
  Demux/53 -> Mux1/29
  Demux/54 -> Mux1/30
  Demux/55 -> Mux1/31
  Demux/56 -> Mux1/32
  Demux/57 -> Mux1/33
  Demux/58 -> Mux1/34
  Demux/59 -> Mux1/35
  Demux/60 -> Mux1/36
  Demux/61 -> Mux1/37
  Demux/62 -> Mux1/38
  Demux/63 -> Mux1/39
  Demux/64 -> Mux1/40
  Demux/65 -> Mux1/41
  Demux/66 -> Mux1/42
  Demux/67 -> Mux1/43
  Demux/68 -> Mux1/44
  Demux/69 -> Mux1/45
  Demux/70 -> Mux1/46
  Demux/71 -> Mux1/47
  Demux/72 -> Mux1/48
  Demux/73 -> Mux1/49
  Demux/74 -> Mux1/50
  Demux/75 -> Mux1/51
  Demux/76 -> Mux1/52
  Demux/77 -> Mux1/53
  Demux/78 -> Mux1/54
  Demux/79 -> Mux1/55
  Demux/80 -> Mux1/56
  Demux/81 -> Mux1/57
  Demux/82 -> Mux1/58
  Demux/83 -> Mux1/59
  Demux/84 -> Mux1/60
  Demux/85 -> Mux1/61
  Demux/86 -> Mux1/62
  Demux/87 -> Mux1/63
  Demux/88 -> Mux1/64
  Demux/89 -> Mux1/65
  Demux/90 -> Mux1/66
  Demux/91 -> Mux1/67
  Demux/92 -> Mux1/68
  Demux/93 -> Mux1/69
  Demux/94 -> Mux1/70
  Demux/95 -> Mux1/71
  Demux/96 -> Mux1/72
  Demux/97 -> Mux1/73
  Demux/98 -> Mux1/74
  Demux/99 -> Mux1/75
  Demux/100 -> Mux1/76
  Mux1/1 -> Terminator/1
  In1/1 -> Bus Selector/1
  Bus Selector/1 -> Demux/1  "<Bal_Cmd>"

== system Controller_HIL/CAN Rx/RX_FIFO_Complete_Event ==
  ID : Inport
  Data : Inport  Port=2
  function : TriggerPort  TriggerType=function-call  VariantControl=Variant
  Temperature : Subsystem
  Voltage : Subsystem
  Pack_Current : Outport
  SRE_uint : Outport  Port=2
  Cell_Temperatures : Outport  Port=3
  Cell_Voltages_76Cells : Outport  Port=4
  wires:
  Data/1 -> Temperature/2(Data), Voltage/2(Data)
  Temperature/1(Outport) -> Pack_Current/1
  Temperature/2(Outport1) -> SRE_uint/1
  Temperature/3(Out3) -> Cell_Temperatures/1
  ID/1 -> Voltage/1(ID), Temperature/1(In1)
  Voltage/1(Voltage_76Cells) -> Cell_Voltages_76Cells/1

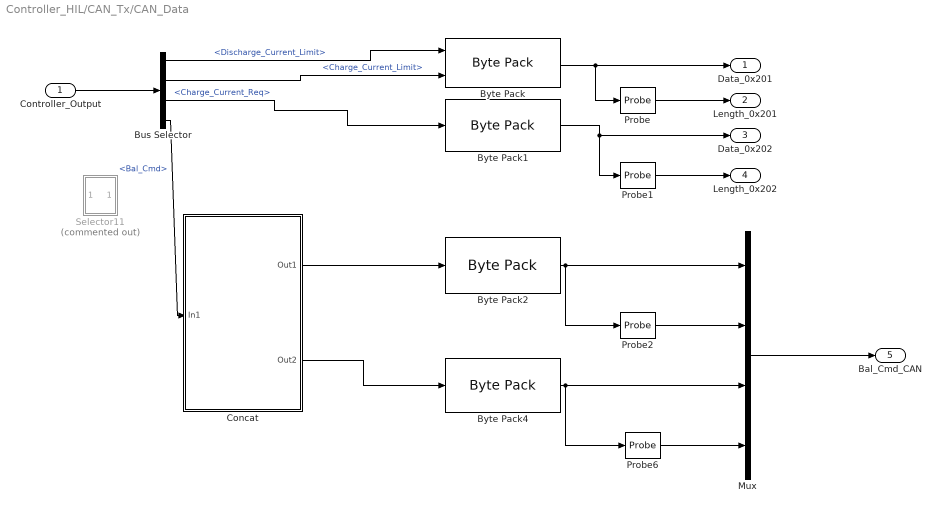
== system Controller_HIL/CAN_Tx/CAN_Data ==
  Controller_Output : Inport
  Bus Selector : BusSelector  OutputSignals=Discharge_Current_Limit,Charge_Current_Limit,Charge_Current_Req,Bal_Cmd
  Byte Pack : etargetslib/Byte Pack  datatypes={'single','single'}  byteAlign=1
  Byte Pack1 : etargetslib/Byte Pack  datatypes={'single'}  byteAlign=1
  Byte Pack2 : etargetslib/Byte Pack  datatypes={'uint8'}  byteAlign=1
  Byte Pack4 : etargetslib/Byte Pack  datatypes={'uint8'}  byteAlign=1
  Concat : Subsystem
  Mux : Mux
  Probe{,1..2,6} (4 alike) : Probe  ProbeSampleTime=off  ProbeComplexSignal=off  ProbeWidthDataType=Same as input
  Selector11 : Subsystem  Commented=on
  Data_0x201 : Outport
  Length_0x201 : Outport  Port=2
  Data_0x202 : Outport  Port=3
  Length_0x202 : Outport  Port=4
  Bal_Cmd_CAN : Outport  Port=5
  wires:
  Bus Selector/3 -> Byte Pack1/1  "<Charge_Current_Req>"
  Controller_Output/1 -> Bus Selector/1
  Probe/1 -> Length_0x201/1
  Byte Pack/1 -> Probe/1, Data_0x201/1
  Byte Pack1/1 -> Probe1/1, Data_0x202/1
  Probe1/1 -> Length_0x202/1
  Bus Selector/1 -> Byte Pack/1  "<Discharge_Current_Limit>"
  Bus Selector/2 -> Byte Pack/2  "<Charge_Current_Limit>"
  Bus Selector/4 -> Concat/1(In1)  "<Bal_Cmd>"
  Byte Pack2/1 -> Probe2/1, Mux/1
  Byte Pack4/1 -> Probe6/1, Mux/3
  Probe2/1 -> Mux/2
  Probe6/1 -> Mux/4
  Mux/1 -> Bal_Cmd_CAN/1
  Concat/1(Out1) -> Byte Pack2/1
  Concat/2(Out2) -> Byte Pack4/1

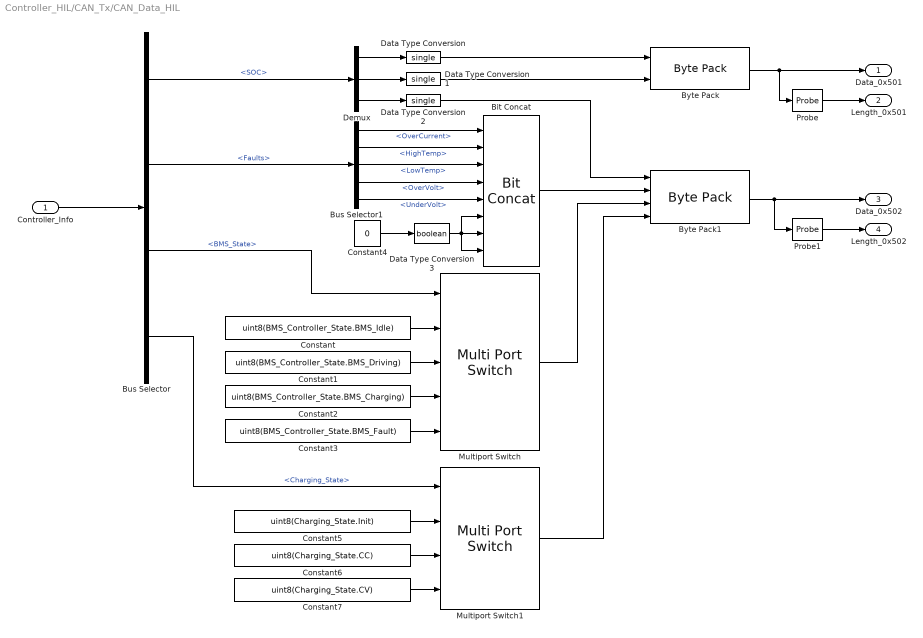
== system Controller_HIL/CAN_Tx/CAN_Data_HIL ==
  Controller_Info : Inport
  Bit Concat : hdlsllib/Logic and Bit Operations/Bit Concat  numInputs=8
  Bus Selector : BusSelector  OutputSignals=SOC,Faults,BMS_State,Charging_State
  Bus Selector1 : BusSelector  OutputSignals=OverCurrent,HighTemp,LowTemp,OverVolt,UnderVolt
  Byte Pack : etargetslib/Byte Pack  datatypes={'single','single'}  byteAlign=1
  Byte Pack1 : etargetslib/Byte Pack  datatypes={'single','uint8','uint8','uint8'}  byteAlign=1
  Constant : Constant  Value=uint8(BMS_Controller_State.BMS_Idle)  SampleTime=-1
  Constant1 : Constant  Value=uint8(BMS_Controller_State.BMS_Driving)  SampleTime=-1
  Constant2 : Constant  Value=uint8(BMS_Controller_State.BMS_Charging)  SampleTime=-1
  Constant3 : Constant  Value=uint8(BMS_Controller_State.BMS_Fault)  SampleTime=-1
  Constant4 : Constant  Value=0  SampleTime=-1
  Constant5 : Constant  Value=uint8(Charging_State.Init)  SampleTime=-1
  Constant6 : Constant  Value=uint8(Charging_State.CC)  SampleTime=-1
  Constant7 : Constant  Value=uint8(Charging_State.CV)  SampleTime=-1
  Data Type Conversion : DataTypeConversion  OutDataTypeStr=single  SaturateOnIntegerOverflow=off  RndMeth=Floor
  Data Type Conversion1 : DataTypeConversion  OutDataTypeStr=single  SaturateOnIntegerOverflow=off  RndMeth=Floor
  Data Type Conversion2 : DataTypeConversion  OutDataTypeStr=single  SaturateOnIntegerOverflow=off  RndMeth=Floor
  Data Type Conversion3 : DataTypeConversion  OutDataTypeStr=boolean  SaturateOnIntegerOverflow=off  RndMeth=Floor
  Demux : Demux  Outputs=3
  Multiport Switch : MultiPortSwitch  DataPortOrder=Specify indices  DataPortIndices={BMS_Controller_State.BMS_Idle, BMS_Controller_State.BMS_Driving, BMS_Controller_State.BMS_Charging, BMS_Controller_State.BMS_Fault}  OutDataTypeStr=uint8  SaturateOnIntegerOverflow=off  InputSameDT=off
  Multiport Switch1 : MultiPortSwitch  DataPortOrder=Specify indices  DataPortIndices={Charging_State.Init, Charging_State.CC, Charging_State.CV}  OutDataTypeStr=uint8  SaturateOnIntegerOverflow=off  InputSameDT=off
  Probe : Probe  ProbeSampleTime=off  ProbeComplexSignal=off  ProbeWidthDataType=Same as input
  Probe1 : Probe  ProbeSampleTime=off  ProbeComplexSignal=off  ProbeWidthDataType=Same as input
  Data_0x501 : Outport
  Length_0x501 : Outport  Port=2
  Data_0x502 : Outport  Port=3
  Length_0x502 : Outport  Port=4
  wires:
  Controller_Info/1 -> Bus Selector/1
  Probe/1 -> Length_0x501/1
  Byte Pack/1 -> Probe/1, Data_0x501/1
  Byte Pack1/1 -> Data_0x502/1, Probe1/1
  Probe1/1 -> Length_0x502/1
  Constant/1 -> Multiport Switch/2
  Constant1/1 -> Multiport Switch/3
  Constant2/1 -> Multiport Switch/4
  Constant3/1 -> Multiport Switch/5
  Demux/1 -> Data Type Conversion/1
  Demux/2 -> Data Type Conversion1/1
  Data Type Conversion/1 -> Byte Pack/1
  Data Type Conversion1/1 -> Byte Pack/2
  Demux/3 -> Data Type Conversion2/1
  Bit Concat/1 -> Byte Pack1/2
  Multiport Switch/1 -> Byte Pack1/3
  Data Type Conversion2/1 -> Byte Pack1/1
  Bus Selector/1 -> Demux/1  "<SOC>"
  Bus Selector/2 -> Bus Selector1/1  "<Faults>"
  Bus Selector/3 -> Multiport Switch/1  "<BMS_State>"
  Bus Selector1/1 -> Bit Concat/1  "<OverCurrent>"
  Bus Selector1/2 -> Bit Concat/2  "<HighTemp>"
  Bus Selector1/3 -> Bit Concat/3  "<LowTemp>"
  Bus Selector1/4 -> Bit Concat/4  "<OverVolt>"
  Bus Selector1/5 -> Bit Concat/5  "<UnderVolt>"
  Constant4/1 -> Data Type Conversion3/1
  Data Type Conversion3/1 -> Bit Concat/8, Bit Concat/6, Bit Concat/7
  Constant5/1 -> Multiport Switch1/2
  Constant7/1 -> Multiport Switch1/4
  Constant6/1 -> Multiport Switch1/3
  Bus Selector/4 -> Multiport Switch1/1  "<Charging_State>"
  Multiport Switch1/1 -> Byte Pack1/4

== system Controller_HIL/CAN_Tx/TX_Complete_HIL ==
  Data_0x501 : Inport
  Length_0x501 : Inport  Port=2
  Data_0x502 : Inport  Port=3
  Length_0x502 : Inport  Port=4
  FCAN_Send_ID_0x501 : mbd_s32k1xx_ec_toolbox/Communication Blocks/CAN Blocks/FCAN_Send  Priority=2  can_instance=0  can_mode=Non-blocking  can_timeout_ms=0  can_mb_idx=18  can_mb_init=Once  show_id_input=off  can_extended_id=off  can_is_remote=off  can_id=501  show_adv_opts=on  can_fd_enable=off  can_enable_brs=off  can_fd_padding=0
  FCAN_Send_ID_0x502 : mbd_s32k1xx_ec_toolbox/Communication Blocks/CAN Blocks/FCAN_Send  Priority=2  can_instance=0  can_mode=Non-blocking  can_timeout_ms=0  can_mb_idx=19  can_mb_init=Once  show_id_input=off  can_extended_id=off  can_is_remote=off  can_id=502  show_adv_opts=on  can_fd_enable=off  can_enable_brs=off  can_fd_padding=0
  wires:
  Length_0x502/1 -> FCAN_Send_ID_0x502/2
  Data_0x502/1 -> FCAN_Send_ID_0x502/1
  Data_0x501/1 -> FCAN_Send_ID_0x501/1
  Length_0x501/1 -> FCAN_Send_ID_0x501/2

== system Controller_HIL/CAN_Tx/Tx_Complete ==
  Data_0x201 : Inport
  Length_0x201 : Inport  Port=2
  Data_0x202 : Inport  Port=3
  Length_0x202 : Inport  Port=4
  Bal_Cmd_CAN : Inport  Port=5
  Demux : Demux
  FCAN_Send_ID_0x1 : mbd_s32k1xx_ec_toolbox/Communication Blocks/CAN Blocks/FCAN_Send  Priority=2  can_instance=0  can_mode=Non-blocking  can_timeout_ms=0  can_mb_idx=0  can_mb_init=Once  show_id_input=off  can_extended_id=off  can_is_remote=off  can_id=203  show_adv_opts=on  can_fd_enable=off  can_enable_brs=off  can_fd_padding=0
  FCAN_Send_ID_0x2 : mbd_s32k1xx_ec_toolbox/Communication Blocks/CAN Blocks/FCAN_Send  Priority=2  can_instance=0  can_mode=Non-blocking  can_timeout_ms=0  can_mb_idx=1  can_mb_init=Once  show_id_input=off  can_extended_id=off  can_is_remote=off  can_id=204  show_adv_opts=on  can_fd_enable=off  can_enable_brs=off  can_fd_padding=0
  FCAN_Send_ID_0x201 : mbd_s32k1xx_ec_toolbox/Communication Blocks/CAN Blocks/FCAN_Send  Priority=2  can_instance=0  can_mode=Non-blocking  can_timeout_ms=0  can_mb_idx=16  can_mb_init=Once  show_id_input=off  can_extended_id=off  can_is_remote=off  can_id=201  show_adv_opts=on  can_fd_enable=off  can_enable_brs=off  can_fd_padding=0
  FCAN_Send_ID_0x202 : mbd_s32k1xx_ec_toolbox/Communication Blocks/CAN Blocks/FCAN_Send  Priority=2  can_instance=0  can_mode=Non-blocking  can_timeout_ms=0  can_mb_idx=17  can_mb_init=Once  show_id_input=off  can_extended_id=off  can_is_remote=off  can_id=202  show_adv_opts=on  can_fd_enable=off  can_enable_brs=off  can_fd_padding=0
  wires:
  Length_0x202/1 -> FCAN_Send_ID_0x202/2
  Data_0x202/1 -> FCAN_Send_ID_0x202/1
  Data_0x201/1 -> FCAN_Send_ID_0x201/1
  Length_0x201/1 -> FCAN_Send_ID_0x201/2
  Demux/4 -> FCAN_Send_ID_0x2/2
  Demux/3 -> FCAN_Send_ID_0x2/1
  Demux/2 -> FCAN_Send_ID_0x1/2
  Demux/1 -> FCAN_Send_ID_0x1/1
  Bal_Cmd_CAN/1 -> Demux/1

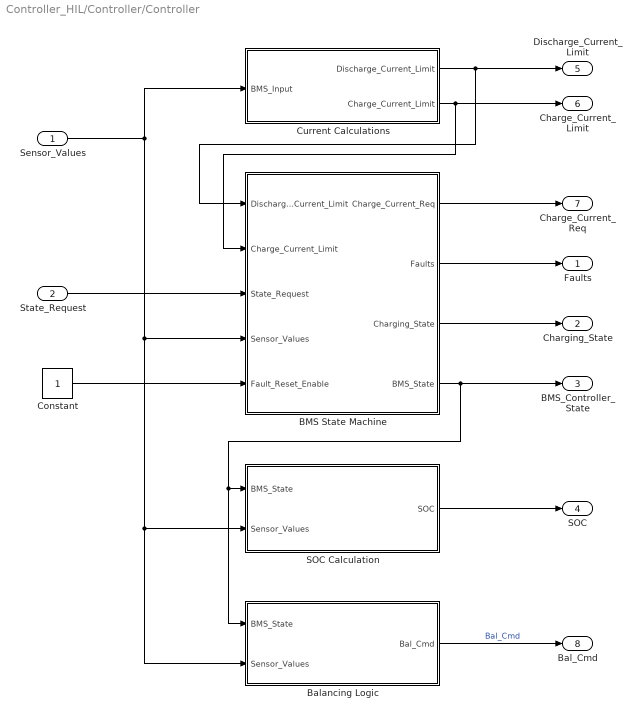
== system Controller_HIL/Controller/Controller ==
  Sensor_Values : Inport  OutDataTypeStr=Bus: Sensor_Values  BusOutputAsStruct=on
  State_Request : Inport  Port=2  OutDataTypeStr=Enum: SRE  PortDimensions=1
  BMS State Machine : Subsystem
  Balancing Logic : Subsystem
  Constant : Constant
  Current Calculations : Subsystem
  SOC Calculation : Subsystem
  Faults : Outport
  Charging_State : Outport  Port=2
  BMS_Controller_State : Outport  Port=3
  SOC : Outport  Port=4
  Discharge_Current_Limit : Outport  Port=5
  Charge_Current_Limit : Outport  Port=6
  Charge_Current_Req : Outport  Port=7
  Bal_Cmd : Outport  Port=8
  wires:
  SOC Calculation/1(SOC) -> SOC/1
  Current Calculations/1(Discharge_Current_Limit) -> BMS State Machine/1(Discharge_Current_Limit), Discharge_Current_Limit/1
  BMS State Machine/2(Faults) -> Faults/1
  BMS State Machine/1(Charge_Current_Req) -> Charge_Current_Req/1
  Sensor_Values/1 -> Balancing Logic/2(Sensor_Values), SOC Calculation/2(Sensor_Values), BMS State Machine/4(Sensor_Values), Current Calculations/1(BMS_Input)
  BMS State Machine/4(BMS_State) -> BMS_Controller_State/1, Balancing Logic/1(BMS_State), SOC Calculation/1(BMS_State)
  Current Calculations/2(Charge_Current_Limit) -> BMS State Machine/2(Charge_Current_Limit), Charge_Current_Limit/1
  Balancing Logic/1(Bal_Cmd) -> Bal_Cmd/1  "Bal_Cmd"
  State_Request/1 -> BMS State Machine/3(State_Request)
  Constant/1 -> BMS State Machine/5(Fault_Reset_Enable)
  BMS State Machine/3(Charging_State) -> Charging_State/1
